simulink model "lab62"  (Simulink 8.0)
settings: Solver=ode45  StartTime=0.0  StopTime=10.0  RelTol=1e-3
libraries: commdigbbndpm3 x4, commchan3 x2, commsink2 x2, commrandsrc2 x1
settings Model: Creator=Dimav  LastModifiedBy=Dimav

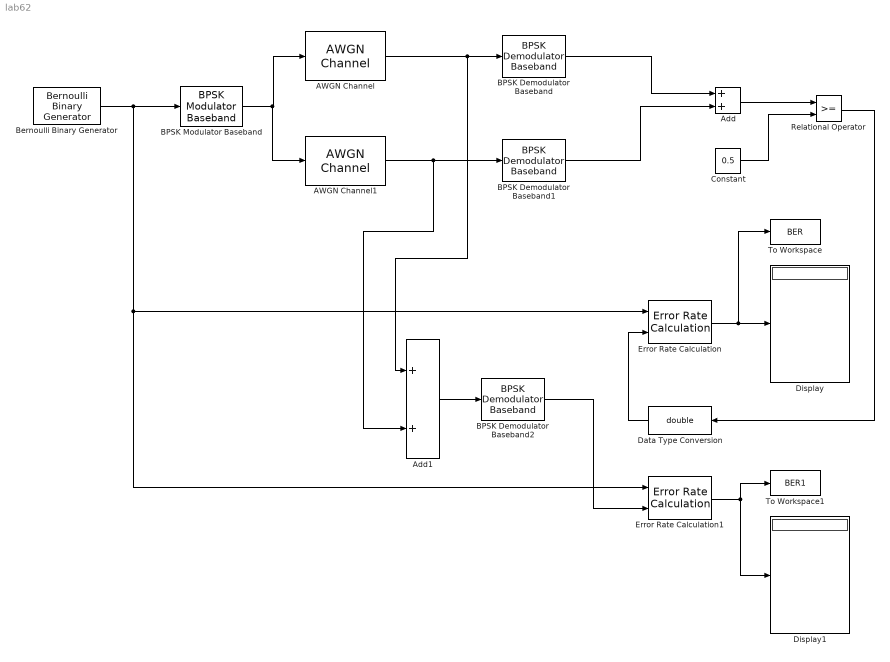
== system lab62 ==
  AWGN Channel : commchan3/AWGN Channel  InputProcessing=Columns as channels (frame based)  seed=67  noiseMode="Signal to noise ratio  (Eb/No)"  EbNodB=3  EsNodB=10  SNRdB=10  bitsPerSym=1  Ps=1  Tsym=1/1200  variance=1
  AWGN Channel1 : commchan3/AWGN Channel  InputProcessing=Columns as channels (frame based)  seed=67  noiseMode="Signal to noise ratio  (Eb/No)"  EbNodB=10  EsNodB=10  SNRdB=10  bitsPerSym=1  Ps=1  Tsym=1/1200  variance=1
  Add : Sum
  Add1 : Sum
  BPSK Demodulator Baseband : commdigbbndpm3/BPSK Demodulator Baseband  Ph=0  DecType=Hard decision  VarSource=Dialog  Variance=1  outDtype=Inherit via internal rule  derotateFactorWordLen=16
  BPSK Demodulator Baseband1 : commdigbbndpm3/BPSK Demodulator Baseband  Ph=0  DecType=Hard decision  VarSource=Dialog  Variance=1  outDtype=Inherit via internal rule  derotateFactorWordLen=16
  BPSK Demodulator Baseband2 : commdigbbndpm3/BPSK Demodulator Baseband  Ph=0  DecType=Hard decision  VarSource=Dialog  Variance=1  outDtype=Inherit via internal rule  derotateFactorWordLen=16
  BPSK Modulator Baseband : commdigbbndpm3/BPSK Modulator Baseband  Ph=0  outDtype=double  outWordLen=16  outUDDataType=sfix(16)  outFracLenMode=Best precision  outFracLen=15
  Bernoulli Binary Generator : commrandsrc2/Bernoulli Binary Generator  P=0.5  seed=61  Ts=1/1200  frameBased=on  sampPerFrame=1  orient=off  outDataType=double
  Constant : Constant  Value=0.5
  Data Type Conversion : DataTypeConversion  OutDataTypeStr=double
  Display : Display
  Display1 : Display
  Error Rate Calculation : commsink2/Error Rate Calculation  N=0  st_delay=0  cp_mode=Entire frame  subframe=[]  PMode=Port  WsName=ErrorVec  RsMode2=off  stop=off  numErr=100  maxBits=1e6
  Error Rate Calculation1 : commsink2/Error Rate Calculation  N=0  st_delay=0  cp_mode=Entire frame  subframe=[]  PMode=Port  WsName=ErrorVec  RsMode2=off  stop=off  numErr=100  maxBits=1e6
  Relational Operator : RelationalOperator  OutDataTypeStr=boolean
  To Workspace : ToWorkspace  VariableName=BER  SampleTime=-1  SaveFormat=Timeseries
  To Workspace1 : ToWorkspace  VariableName=BER1  SampleTime=-1  SaveFormat=Timeseries
  wires:
  Bernoulli Binary Generator/1 -> Error Rate Calculation/1, Error Rate Calculation1/1, BPSK Modulator Baseband/1
  BPSK Modulator Baseband/1 -> AWGN Channel1/1, AWGN Channel/1
  BPSK Demodulator Baseband/1 -> Add/1
  BPSK Demodulator Baseband1/1 -> Add/2
  Constant/1 -> Relational Operator/2
  Add/1 -> Relational Operator/1
  Relational Operator/1 -> Data Type Conversion/1
  Data Type Conversion/1 -> Error Rate Calculation/2
  AWGN Channel1/1 -> Add1/2, BPSK Demodulator Baseband1/1
  AWGN Channel/1 -> Add1/1, BPSK Demodulator Baseband/1
  Add1/1 -> BPSK Demodulator Baseband2/1
  BPSK Demodulator Baseband2/1 -> Error Rate Calculation1/2
  Error Rate Calculation1/1 -> To Workspace1/1, Display1/1
  Error Rate Calculation/1 -> To Workspace/1, Display/1
